simulink model "gm_RaisedCosine"  (R2022a)
settings: Solver=FixedStepDiscrete  StartTime=0.0  StopTime=0.001  FixedStep=1e-9  RelTol=1e-3
libraries: dspmlti4 x2
settings Model: Creator=okoko  LastModifiedBy=okoko
settings OptimizationCC: BlockReduction=off  ConditionallyExecuteInputs=off
settings DebuggingCC: InheritedTsInSrcMsg=none  SingleTaskRateTransMsg=error

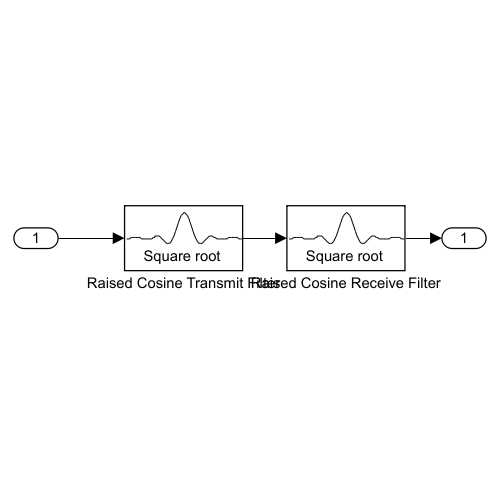
[thumbnail: Simulink's stored preview of the top-level diagram]
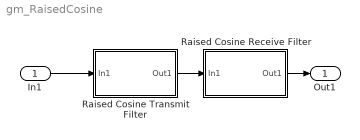
== system gm_RaisedCosine ==
  In1 : Inport  OutMin=-4  OutMax=4  OutDataTypeStr=fixdt(1, 16, 12)  PortDimensions=1  SampleTime=0.1
  Raised Cosine Receive Filter : Subsystem  mask(Raised Cosine Receive Filter){filtType=Square root, R=double(0.2), filtSpan=double(16), N=double(4), downFactor=double(4), downOffset=double(0), filterGain=double(1), InputProcessing=Elements as channels (sample based), RateOptions=Allow multirate processing, framing=Mute, checkCoeff=off, variableName=rcRxFilt, currentFiltSpan=double(10), D=double(5), inputOffset=double(0), sampMode=Mute, saveAsFlag=double(0), rateMode=Downsampling, checkGain=Normalized, launchFVT=on, roundingMode=Floor, overflowMode=off, coeffMode=Same word length as input, coeffWordLength=double(16), coeffFracLength=double(15), coeffDataTypeStr=Inherit: Same word length as input, coeffMin=[], coeffMax=[], coeffLastDataTypeStr=Inherit: Same word length as input, prodOutputMode=Same as input, prodOutputWordLength=double(32), prodOutputFracLength=double(30), prodOutputDataTypeStr=Inherit: Same as input, prodOutputLastDataTypeStr=Inherit: Same as input, accumMode=Same as product output, accumWordLength=double(32), accumFracLength=double(30), accumDataTypeStr=Inherit: Same as product output, accumLastDataTypeStr=Inherit: Same as product output, outputMode=Same as accumulator, outputWordLength=double(16), outputFracLength=double(15), outputDataTypeStr=Inherit: Same as accumulator, outputMin=[], outputMax=[], outputLastDataTypeStr=Inherit: Same as accumulator, LockScale=off}
      mask prompts: filtType "Filter shape:"; R "Rolloff factor:"; filtSpan "Filter span in symbols:"; N "Input samples per symbol:"; downFactor "Decimation factor:"; downOffset "Decimation offset:"; filterGain "Linear amplitude filter gain:"; InputProcessing "dsp:FIRMultirateBlockDialog:InputProc_MP"; RateOptions "dsp:FIRMultirateBlockDialog:RateOptions_MP"; checkCoeff "Export filter coefficients to workspace"; variableName "Coefficient variable name:"; currentFiltSpan "Current filter span in symbols:"; D "Group delay (number of symbols):"; sampMode "Input sampling mode:"; saveAsFlag "Save_as flag:"; rateMode "Output mode:"; checkGain "Filter gain:"; launchFVT "Visualize filter with FVTool"; roundingMode "dspshared:FixptDialog:roundingMode"; overflowMode "Simulink:masks:SaturateOnIntegerOverflow_MP"; LockScale "dspshared:FixptDialog:lockAgnstChanges"
      mask help: Filter the input, and, if selected, downsample, using a normal or square root raised cosine FIR filter.
      mask init:
      | D = double(5);
      | InputProcessing = double(2);
      | LockScale = double(0);
      | N = double(4);
      | R = double(0.2);
      | RateOptions = double(2);
      | accumDataTypeStr = 'Inherit: Same as product output';
      | accumFracLength = double(30);
      | accumLastDataTypeStr = 'Inherit: Same as product output';
      | accumMode = double(1);
      | accumWordLength = double(32);
      | checkCoeff = double(0);
      | checkGain = double(1);
      | coeff = reshape(double([-0.0014581923365742395 0.001676602837942445 0.003638041536615476 0.0026883459298042583 -0.0005837512746960972 -0.003504033820841154 -0.003403238076468691 1.3647689001810081e-17 0.003966465682162914 0.004701064008085029 0.0006440626479794659 -0.0055687165688802845 -0.008488763585436107 -0.004103264840227574 0.00610253409841469 0.014840613829444899 0.01367986143041476 -1.0720603939673657e-17 -0.018968296719058572 -0.029110434819295743 -0.018866737427957365 0.010631186176953255 0.04244381792718055 0.05197468797621584 0.023294581662310503 -0.03604149072865189 -0.09237201012790064 -0.10000588994274985 -0.026274643529296676 0.12614521755028157 0.31357254640918014 0.46777219178594265 0.5273550135525409 0.46777219178594265 0.31357254640918014 0.12614521755028157 -0.026274643529296676 -0.10000588994274985 -0.09237201012790064 -0.03604149072865189 0.023294581662310503 0.05197468797621584 0.04244381792718055 0.010631186176953255 -0.018866737427957365 -0.029110434819295743 -0.018968296719058572 -1.0720603939673657e-17 0.01367986143041476 0.014840613829444899 0.00610253409841469 -0.004103264840227574 -0.008488763585436107 -0.0055687165688802845 0.0006440626479794659 0.004701064008085029 0.003966465682162914 1.3647689001810081e-17 -0.003403238076468691 -0.003504033820841154 -0.0005837512746960972 0.0026883459298042583 0.003638041536615476 0.001676602837942445 -0.0014581923365742395]).', [1  65]);
      | coeffDataTypeStr = 'Inherit: Same word length as input';
      | coeffFracLength = double(15);
      | coeffLastDataTypeStr = 'Inherit: Same word length as input';
      | coeffMax = [];
      | coeffMin = [];
      | coeffMode = double(1);
      | coeffWordLength = double(16);
      | currentFiltSpan = double(10);
      | downFactor = double(4);
      | downOffset = double(0);
      | filtSpan = double(16);
      | filtType = double(2);
      | filterGain = double(1);
      | framing = double(5);
      | inputOffset = double(0);
      | launchFVT = double(1);
      | outputDataTypeStr = 'Inherit: Same as accumulator';
      | outputFracLength = double(15);
      | outputLastDataTypeStr = 'Inherit: Same as accumulator';
      | outputMax = [];
      | outputMin = [];
      | outputMode = double(1);
      | outputWordLength = double(16);
      | overflowMode = double(0);
      | prodOutputDataTypeStr = 'Inherit: Same as input';
      | prodOutputFracLength = double(30);
      | prodOutputLastDataTypeStr = 'Inherit: Same as input';
      | prodOutputMode = double(1);
      | prodOutputWordLength = double(32);
      | rateMode = double(1);
      | roundingMode = double(3);
      | sampMode = double(3);
      | saveAsFlag = double(0);
      | variableName = 'rcRxFilt';
      mask Help: eval('blocksethelp');
      mask TypeOptions filtType: Normal | Square root
      mask TypeOptions InputProcessing: Columns as channels (frame based) | Elements as channels (sample based)
      mask Callback InputProcessing: commblkrcfiltrx(gcbh,'cbInputProcessing');
      mask TypeOptions RateOptions: Enforce single-rate processing | Allow multirate processing
      mask TypeOptions framing: Enforce single-rate processing | Allow multirate processing | Maintain input frame rate | Maintain input frame size | Mute
      mask Callback checkCoeff: commblkrcfiltrx(gcbh,'cbCheckCoeff');
      mask Callback variableName: commblkrcfiltrx(gcbh,'dialogdynamic');
      mask TypeOptions sampMode: Frame-based | Sample-based | Mute
      mask TypeOptions rateMode: Downsampling | None
      mask TypeOptions checkGain: Normalized | User-specified
      mask TypeOptions roundingMode: Ceiling | Convergent | Floor | Nearest | Round | Simplest | Zero
      mask TypeOptions coeffMode: Same word length as input | Specify word length | Binary point scaling | Slope and bias scaling
      mask TypeOptions prodOutputMode: Same as input | Binary point scaling | Slope and bias scaling
      mask TypeOptions accumMode: Same as product output | Same as input | Binary point scaling | Slope and bias scaling
      mask TypeOptions outputMode: Same as accumulator | Same as input | Binary point scaling | Slope and bias scaling
      mask Display:
      | coeffs = rcosdesign(0.2, 10, 8, 'sqrt'); % default
      | % This plot does not change enough to make it worth updating to specifics
      | % Just use a representative plot for all cases.
      | %
      | %-- Init icon variables
      | %   (draw default icon in case of early returns,
      | %    e.g. due to errors from undefined mask params)
      | icon.str = get_param(gcbh,'filtType');
      | icon.x = 0.5;
      | icon.y = 0.25;
      | icon.plot = coeffs/max(coeffs)*0.40+0.50;
      | icon.xx = (1:length(coeffs))/length(coeffs);
      | 
      | plot(0,0,1,1,icon.xx,icon.plot);
      | text(icon.x,icon.y,icon.str,'horiz','center');
  Raised Cosine Transmit Filter : Subsystem  mask(Raised Cosine Transmit Filter){filtType=Square root, R=double(0.2), filtSpan=double(16), N=double(4), filterGain=double(1), InputProcessing=Elements as channels (sample based), RateOptions=Allow multirate processing, framing=Mute, checkCoeff=on, variableName=reshape(double([-0.0014581923365742395 0.001676602837942445 0.003638041536615476 0.0026883459298042583 -0.0005837512746960972 -0.003504033820841154 -0.003403238076468691 1.3647689001810081e-17 0.003966465682162914 0.004701064008085029 0.0006440626479794659 -0.0055687165688802845 -0.008488763585436107 -0.004103264840227574 0.00610253409841469 0.014840613829444899 0.01367986143041476 -1.0720603939673657e-17 -0.018968296719058572 -0.029110434819295743 -0.018866737427957365 0.010631186176953255 0.04244381792718055 0.05197468797621584 0.023294581662310503 -0.03604149072865189 -0.09237201012790064 -0.10000588994274985 -0.026274643529296676 0.12614521755028157 0.31357254640918014 0.46777219178594265 0.5273550135525409 0.46777219178594265 0.31357254640918014 0.12614521755028157 -0.026274643529296676 -0.10000588994274985 -0.09237201012790064 -0.03604149072865189 0.023294581662310503 0.05197468797621584 0.04244381792718055 0.010631186176953255 -0.018866737427957365 -0.029110434819295743 -0.018968296719058572 -1.0720603939673657e-17 0.01367986143041476 0.014840613829444899 0.00610253409841469 -0.004103264840227574 -0.008488763585436107 -0.0055687165688802845 0.0006440626479794659 0.004701064008085029 0.003966465682162914 1.3647689001810081e-17 -0.003403238076468691 -0.003504033820841154 -0.0005837512746960972 0.0026883459298042583 0.003638041536615476 0.001676602837942445 -0.0014581923365742395]).', [1  65]), checkGain=Normalized, sampMode=Mute, saveAsFlag=double(0), currentFiltSpan=double(10), D=double(5), launchFVT=on, roundingMode=Floor, overflowMode=off, coeffMode=Same word length as input, coeffWordLength=double(16), coeffFracLength=double(0), coeffDataTypeStr=Inherit: Same word length as input, coeffMin=[], coeffMax=[], coeffLastDataTypeStr=Inherit: Same word length as input, prodOutputMode=Inherit via internal rule, prodOutputWordLength=double(16), prodOutputFracLength=double(0), prodOutputDataTypeStr=Inherit: Inherit via internal rule, prodOutputLastDataTypeStr=Inherit: Inherit via internal rule, accumMode=Inherit via internal rule, accumWordLength=double(16), accumFracLength=double(0), accumDataTypeStr=Inherit: Inherit via internal rule, accumLastDataTypeStr=Inherit: Inherit via internal rule, outputMode=Same as input, outputWordLength=double(16), outputFracLength=double(0), outputDataTypeStr=Inherit: Same as input, outputMin=[], outputMax=[], outputLastDataTypeStr=Inherit: Same as input, LockScale=off}
      mask prompts: filtType "Filter shape:"; R "Rolloff factor:"; filtSpan "Filter span in symbols:"; N "Output samples per symbol:"; filterGain "Linear amplitude filter gain:"; InputProcessing "dsp:FIRMultirateBlockDialog:InputProc_MP"; RateOptions "dsp:FIRMultirateBlockDialog:RateOptions_MP"; checkCoeff "Export filter coefficients to workspace"; variableName "Coefficient variable name:"; checkGain "Filter gain:"; sampMode "Input sampling mode:"; saveAsFlag "Save_as flag:"; currentFiltSpan "Current filter span in symbols:"; D "Group delay (number of symbols):"; launchFVT "Visualize filter with FVTool"; roundingMode "dspshared:FixptDialog:roundingMode"; overflowMode "Simulink:masks:SaturateOnIntegerOverflow_MP"; LockScale "dspshared:FixptDialog:lockAgnstChanges"
      mask help: Upsample and filter the input signal using a normal or square root raised cosine FIR filter.
      mask init:
      | D = double(5);
      | InputProcessing = double(2);
      | LockScale = double(0);
      | N = double(4);
      | R = double(0.2);
      | RateOptions = double(2);
      | accumDataTypeStr = 'Inherit: Inherit via internal rule';
      | accumFracLength = double(0);
      | accumLastDataTypeStr = 'Inherit: Inherit via internal rule';
      | accumMode = double(1);
      | accumWordLength = double(16);
      | checkCoeff = double(1);
      | checkGain = double(1);
      | coeff = reshape(double([-0.0014581923365742395 0.001676602837942445 0.003638041536615476 0.0026883459298042583 -0.0005837512746960972 -0.003504033820841154 -0.003403238076468691 1.3647689001810081e-17 0.003966465682162914 0.004701064008085029 0.0006440626479794659 -0.0055687165688802845 -0.008488763585436107 -0.004103264840227574 0.00610253409841469 0.014840613829444899 0.01367986143041476 -1.0720603939673657e-17 -0.018968296719058572 -0.029110434819295743 -0.018866737427957365 0.010631186176953255 0.04244381792718055 0.05197468797621584 0.023294581662310503 -0.03604149072865189 -0.09237201012790064 -0.10000588994274985 -0.026274643529296676 0.12614521755028157 0.31357254640918014 0.46777219178594265 0.5273550135525409 0.46777219178594265 0.31357254640918014 0.12614521755028157 -0.026274643529296676 -0.10000588994274985 -0.09237201012790064 -0.03604149072865189 0.023294581662310503 0.05197468797621584 0.04244381792718055 0.010631186176953255 -0.018866737427957365 -0.029110434819295743 -0.018968296719058572 -1.0720603939673657e-17 0.01367986143041476 0.014840613829444899 0.00610253409841469 -0.004103264840227574 -0.008488763585436107 -0.0055687165688802845 0.0006440626479794659 0.004701064008085029 0.003966465682162914 1.3647689001810081e-17 -0.003403238076468691 -0.003504033820841154 -0.0005837512746960972 0.0026883459298042583 0.003638041536615476 0.001676602837942445 -0.0014581923365742395]).', [1  65]);
      | coeffDataTypeStr = 'Inherit: Same word length as input';
      | coeffFracLength = double(0);
      | coeffLastDataTypeStr = 'Inherit: Same word length as input';
      | coeffMax = [];
      | coeffMin = [];
      | coeffMode = double(1);
      | coeffWordLength = double(16);
      | currentFiltSpan = double(10);
      | filtSpan = double(16);
      | filtType = double(2);
      | filterGain = double(1);
      | framing = double(5);
      | launchFVT = double(1);
      | outputDataTypeStr = 'Inherit: Same as input';
      | outputFracLength = double(0);
      | outputLastDataTypeStr = 'Inherit: Same as input';
      | outputMax = [];
      | outputMin = [];
      | outputMode = double(3);
      | outputWordLength = double(16);
      | overflowMode = double(0);
      | prodOutputDataTypeStr = 'Inherit: Inherit via internal rule';
      | prodOutputFracLength = double(0);
      | prodOutputLastDataTypeStr = 'Inherit: Inherit via internal rule';
      | prodOutputMode = double(1);
      | prodOutputWordLength = double(16);
      | rateFactor = double(4);
      | roundingMode = double(3);
      | sampMode = double(3);
      | saveAsFlag = double(0);
      | variableName = 'rcTxFilt';
      mask Help: eval('blocksethelp');
      mask TypeOptions filtType: Normal | Square root
      mask TypeOptions InputProcessing: Columns as channels (frame based) | Elements as channels (sample based)
      mask Callback InputProcessing: commblkrcfilttx(gcbh,'cbInputProcessing');
      mask TypeOptions RateOptions: Enforce single-rate processing | Allow multirate processing
      mask TypeOptions framing: Enforce single-rate processing | Allow multirate processing | Maintain input frame rate | Maintain input frame size | Mute
      mask Callback checkCoeff: commblkrcfilttx(gcbh,'cbCheckCoeff');
      mask Callback variableName: commblkrcfilttx(gcbh,'dialogdynamic');
      mask TypeOptions checkGain: Normalized | User-specified
      mask TypeOptions sampMode: Frame-based | Sample-based | Mute
      mask TypeOptions roundingMode: Ceiling | Convergent | Floor | Nearest | Round | Simplest | Zero
      mask TypeOptions coeffMode: Same word length as input | Specify word length | Binary point scaling | Slope and bias scaling
      mask TypeOptions prodOutputMode: Inherit via internal rule | Same as input | Binary point scaling | Slope and bias scaling
      mask TypeOptions accumMode: Inherit via internal rule | Same as product output | Same as input | Binary point scaling | Slope and bias scaling
      mask TypeOptions outputMode: Same as accumulator | Same as product output | Same as input | Binary point scaling | Slope and bias scaling
      mask Display:
      | coeffs = rcosdesign(0.2, 10, 8, 'sqrt'); % default
      | % This plot does not change enough to make it worth updating to specifics
      | % Just use a representative plot for all cases.
      | %
      | %-- Init icon variables
      | %   (draw default icon in case of early returns,
      | %    e.g. due to errors from undefined mask params)
      | icon.str = get_param(gcbh,'filtType');
      | icon.x = 0.5;
      | icon.y = 0.25;
      | icon.plot = coeffs/max(coeffs)*0.40+0.50;
      | icon.xx = (1:length(coeffs))/length(coeffs);
      | 
      | plot(0,0,1,1,icon.xx,icon.plot);
      | text(icon.x,icon.y,icon.str,'horiz','center');
  Out1 : Outport  OutMin=-4  OutMax=4  OutDataTypeStr=fixdt(1,16,12)  SampleTime=0.1
  wires:
  In1/1 -> Raised Cosine Transmit Filter/1(In1)
  Raised Cosine Receive Filter/1(Out1) -> Out1/1
  Raised Cosine Transmit Filter/1(Out1) -> Raised Cosine Receive Filter/1(In1)

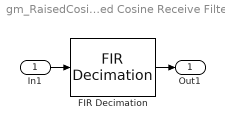
== system gm_RaisedCosine/Raised Cosine Receive Filter ==
  In1 : Inport  OutDataTypeStr=fixdt(1, 16, 12)  SampleTime=0.025
  FIR Decimation : dspmlti4/FIR Decimation  FilterSource=Dialog parameters  h=coeff  D=downFactor  filtStruct=Direct form  FilterObject=Hm_firdecim  framing=Allow multirate processing  inputOffset=(downFactor-downOffset)  outputBufInitCond=0  roundingMode=Floor  overflowMode=off  firstCoeffDataTypeStr=Inherit: Same word length as input  firstCoeffMin=[]  firstCoeffMax=[]  firstCoeffLastDataTypeStr=Inherit: Same word length as input  accumDataTypeStr=Inherit: Same as product output  accumLastDataTypeStr=Inherit: Same as product output  outputDataTypeStr=Inherit: Same as accumulator  outputMin=[]  outputMax=[]  outputLastDataTypeStr=Inherit: Same as accumulator
  Out1 : Outport  SampleTime=0.1
  wires:
  In1/1 -> FIR Decimation/1
  FIR Decimation/1 -> Out1/1

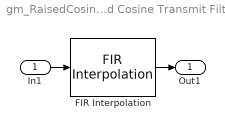
== system gm_RaisedCosine/Raised Cosine Transmit Filter ==
  In1 : Inport  OutDataTypeStr=fixdt(1, 16, 12)  SampleTime=0.1
  FIR Interpolation : dspmlti4/FIR Interpolation  FilterSource=Dialog parameters  PrivateCoeffs=0  h=coeff  L=rateFactor  FilterObject=Hm_firinterp  framing=Allow multirate processing  outputBufInitCond=0  roundingMode=Floor  overflowMode=off  firstCoeffDataTypeStr=Inherit: Same word length as input  firstCoeffMin=[]  firstCoeffMax=[]  firstCoeffLastDataTypeStr=Inherit: Same word length as input  outputMin=[]  outputMax=[]
  Out1 : Outport  SampleTime=0.025
  wires:
  In1/1 -> FIR Interpolation/1
  FIR Interpolation/1 -> Out1/1
